simulink model "CAVE_MachE_speedTrack0202"  (R2019b)
settings: configuration reference "ConfigSetDesktopFixedStep" (kept outside this file)
PreLoadFcn:
  | VSS_BICYCLE=Simulink.Variant('Dual=0');
  | VSS_DUAL=Simulink.Variant('Dual=1');
  | Dual=1;
  | load('DriveCycle2.mat')
PostLoadFcn:
  | if any(exist('dsrtsu_mdlpostloadfcn', 'file') ~= 0), dsrtsu_mdlpostloadfcn('Execute', bdroot); end
InitFcn:
  | , if any(exist('dsmpb_private', 'file') ~= 0), dsmpb_private('dsmpb_mdlclblib', 'Init', bdroot); end,
  | load('DriveCycle2.mat')
model workspace (MAT data in the model file):
  Gas = 0.383333333333
values from neighbouring files (symbols this model uses):
  CoastDown =     [Run_Simulink.mat]
  limitedMCT =     [Run_Simulink.mat]
  MCT =     [Run_Simulink.mat]
  pMCT =     [Run_Simulink.mat]
  Ref_speed = [13 13.007895099 13.015778396 13.023649891 13.031509584 13.039357475 13.047193564 13.055017851 13.062830336 13.070631019 13.0784199 13.086196979 ... (2669 elements, 2669x1)]    [Ref_speed_and_time.mat]
  Ref_time = [0 0.01 0.02 0.03 0.04 0.05 0.06 0.07 0.08 0.09 0.1 0.11 ... (2669 elements, 2669x1)]    [Ref_speed_and_time.mat]
  US06 =     [Run_Simulink.mat]
undefined symbols (not defined in the file or in its folder): AccelCmd, ActTqLF_Nm_, ActTqLR_Nm_, ActTqRF_Nm_, ActTqRR_Nm_, BattChargeLimitMaxPwr, BattChargeLimitSocBpts, BattChargeLimitTbl, BattChrgCapcty, BattDischargeLimitSocBpts, BattDischargeLimitTbl, BattDischargeMaxPwr, BattNumCellsParallel, BattNumCellsSeries, BattOpenVoltCapBpts, BattOpenVoltTbl, BattResistSocBpts, BattResistTbl, BattResistTempBpts, BrakeMaxPrs, BrakeMaxTrq, ChassisDistCg2FrontAxle, ChassisDistCg2RearAxle, ChassisVehMass, CltchCmd, DecelCmd, DiffRatio, DiscIntNeverNeededParam, EnvGravCnst, EnvPrs, EnvTemp, FuelSpecificGrav, GearCmd, h, InitStates, lgSw, MtrEffSpdBpts, MtrEffTbl, MtrEffTrqBpts, MtrPwrMax, MtrTrqMax, Ref_Spd0229, Ref_Time0229, SteeringCmd, SupvsryCtrlRegenBrkCutOffTbl, SupvsryCtrlRegenSpdBpts, TestScnrioCycleNum, VEH
libraries: VSIGenLib x67, simulink x57, etargetslib x38, dsmpblib x28, vehdynlibtire x12, autolibshared x9, vehdynlibsuspension x7, vehdynlibtirecommon x7, autolibutils x5, CarMaker4SL x4, VsrLibWheel x4, autolibpowerinfoutils x3
(part 1 of 14)
PreSaveFcn:
  | , if any(exist('dsmpb_private', 'file') ~= 0), dsmpb_private('dsmpb_mdlclblib', 'PreSave', bdroot); end,
CloseFcn:
  | , if any(exist('dsmpb_private', 'file') ~= 0), dsmpb_private('dsmpb_mdlclblib', 'Close', bdroot); end,
settings Model: DataDictionary=DdPassengerEv.sldd  EnableAccessToBaseWorkspace=off  DSMPB_ID_DATA={'17923',struct('BlockId','31b0f37e-04c7-4ce1-8b16-8a1e9b5cfa15','SignalIds',{{'17c721c6-a3ae-4ad4-b238-642b1de755b7'}}),'17924',struct('BlockId','bcfd9437-88e4-4cd6-b7b0-947b12d9129e','SignalIds',{{'e279c9ec-6196-4878-b889-71a854f53d02'}}),'17925',struct('BlockId','c62c3796-2ab1-49a7-b1e5-4d980e0bcb0b','SignalIds',{{'f66872c7-5266-4e77-ba9d-87065806d94f'}}),'17926',struct('BlockId','40b2dd3c-dc50-4d54-adc2-8ba9b18f36d5','SignalIds',{{'523e7fc5-5d31-4807-939d-dbbffd70444f'}}),'17927',struct('BlockId','e8d674f4-c081-4c3a-b2b1-2d0ab8133194','SignalIds',{{'0eda9826-4c02-4cc0-9f18-cf69c46de25a','ab39894a-9bf0-4e2b-9c49-db18f6b4bbcb','ed4e635a-610c-4130-b876-996df8d6f23e','d7b08fa0-5164-4c6c-899c-f7c626698d6c','66095545-3d28-434a-a0e8-d46feba78e3b'}}),'17928',struct('BlockId','74aeb7d1-659c-488e-9138-a7590a989d80','SignalIds',{{'26f36065-db9f-4eb5-8bd7-2ab8ed1530af','9b8b33d1-0c3b-4425-9130-99ff6edfa98a'}}),'17929',struct('BlockId','1e8a7d48-41ff-4223-b4b4-ccd9c4207a27','SignalIds',{{'1b0cf8dd-8605-4169-a6de-39231325f0e5'}}),'17935',struct('BlockId','a5f9a6b1-85ee-410c-8934-50052dbd8ca7','SignalIds',{{'ba3b2526-034b-43f6-a555-dff2bea2cc85'}}),'17936',struct('BlockId','1e1892f8-2999-45dd-a8da-0e8121fc388b','SignalIds',{{'4c47874d-0703-4ff1-9abe-c2ce178ef0a7'}}),'17937',struct('BlockId','e85c17ff-dd30-482c-995d-c0a74f106bb8','SignalIds',{{'8160658a-6bed-4f87-b995-d0b653e3718e'}}),'17938',struct('BlockId','e3071f67-61ca-4ccc-876b-23b50e94809a','SignalIds',{{'03fc8176-d730-4c60-914d-7ce6c370162b'}}),'17939',struct('BlockId','6cc6af10-99b5-45df-ab2c-9d119c31698c','SignalIds',{{'65b90dff-5318-4540-88c9-38859f061b45'}}),'17940',struct('BlockId','0db74d10-8518-4861-b223-fb8645ae7c50','SignalIds',{{'f8b55a51-0374-486e-9c03-7d81119e1378'}}),'17941',struct('BlockId','43054e70-1d94-41e4-ae6d-92ba2dcfefa2','SignalIds',{{'310153da-09e7-4a32-aa01-e5bac30a61fd'}}),'17942',struct('BlockId','d4d6f3b7-e9bb-4bfb-ad6d-7b0539ed1dac','SignalIds',{{'32f338f5-3495-4abe-a586-ce83ab37ca6d'}}),'18088',struct('BlockId','f88c42c2-e70e-4436-bd85-ff34452e836e','SignalIds',{{'1df572a0-f117-4729-9091-2c1a0a26ec90','0824b86c-995c-4624-95de-4f5a118cf0f7','1af539eb-325a-4e38-9107-84d6b0267392','ebb0fa34-559f-4fe0-b409-8a817ae8753c','d7145080-d35d-4c02-8c9e-cf76ffb14dc2','5075bfde-4142-4aeb-b309-025b37120541','abbab0bd-1456-4252-a37b-ee5f55ea0579','b5d617b8-bb24-4539-9145-e591a0a295f8','7df03788-1936-4801-98c0-dd7f6dfcacba','19949bfb-f246-4995-90e8-29a3751a0fa7','9454b59a-aedd-4270-89a6-1cca43305823','37cf720c-23c2-4b6d-8589-7b035c806643','98db9f76-eafd-4d54-90d2-d997d73b87d4','ff589fc8-5b21-4798-a75e-d26fc35c1fa1','e61b2882-e27e-4f06-b730-5e5281621b34','6605e0e6-8bf3-4a45-a0b0-4b9c1cf463f3','0d0f5161-daad-47a1-bb1d-ec2adbc183ca','48ba6675-0966-4a1c-b127-4f76dca3de94','3c897f11-b2eb-4eb8-b88f-7b7e913c6e41','378f468e-364f-43c5-91f9-fc8ddef6aca6','9c7f20ac-956d-4c19-bdea-31a2a3930ea2','bc252920-9c7c-4b91-a017-ee1d69e3f03c','a5e7a104-8664-4690-a58a-7cbf05737866','fe1cfa34-9b23-4225-85e3-0403f07d36e7','ab40d80a-815e-4994-aacd-e42d283f5b3a','2a4143b2-c438-4d42-997d-0587141eb8f0','2686c37a-8724-40b3-99fb-f8873ba286b8','3707aa1b-88c1-4f14-8f25-f346aa75c252','7413af4b-f834-4020-ad34-3dd98c546e0c','3445835b-9a90-4408-a32d-d76b66b0385b','23c9a144-1259-4fa3-9a16-4a32a7eadff9','5b4206b0-ea89-4111-86f7-7a4fd8c76b72','85c84ea6-72b6-4ccb-9199-727b305580c3','97bb0073-9d03-44a9-972d-49a0eb465678','8c3f0698-b0b6-4624-aa00-3a3096f7cc2f','c968922f-253e-433f-ad46-daf21e902962','21ad150a-19dc-415b-bc1b-b39528ec9221','a3572415-9467-4ff8-a492-c6c1b3cb1b64','700ac678-fb53-40b6-8e97-9eeffe7a1ca8','14ed5f8b-aa1d-402b-b493-5622a729893d','bdbcc0b3-c6a4-485e-8fbf-8c12a8df89e7','7a19cc2b-f06b-466f-ae52-fb8ac6fb0258','87deda6a-2251-4462-8ae0-a20845c776d4','41874d9b-304a-4265-a3a1-69d5c58383ea'}}),'18175',struct('BlockId','8445dc7e-f46b-4bf1-918c-6ff4bf4b4269','SignalIds',{{'24a6103b-da21-4c61-bcdd-b18edd3e31e0'}}),'18251',struct('BlockId','87dadb4f-598f-4630-a764-aa9dbd54dbe2','SignalIds',{{'83e82515-562b-4cea-9022-e0067df93a7f','d6888abe-93df-4986-aa37-664290aa1833','c6c9ff24-fc0f-4a39-be02-e6acd6045705','d4d14bee-f141-4067-bca8-9bf015562c80','1613add9-a5cb-4969-b219-0bfd270ce741'}}),'18719',struct('BlockId','79daabbd-4df4-4017-ba65-d977f7e6cd2f','SignalIds',{{'63c99320-3a8a-469e-8a50-5c577229603f'}}),'18720',struct('BlockId','9f21d727-31d5-41b9-aed1-27a40d8edf8b','SignalIds',{{'abab19c9-0d91-46eb-acba-2a4710e305d8'}}),'18721',struct('BlockId','5513e588-accc-447f-8233-209349c29c53','SignalIds',{{'cf7c35a9-6bda-4f5f-bfb5-f51ad44c376b'}}),'18722',struct('BlockId','a427ee23-ff95-4a9c-807f-ad2b61c33ee4','SignalIds',{{'b3e368f1-9670-4dd7-aa42-1fcccca64ddf'}}),'18723',struct('BlockId','53805a71-03ad-4b45-a2ab-66e4ec3700d0','SignalIds',{{'0801da20-d997-46db-8512-e37e1180e77c','d193450d-1a5a-4c8d-a2ac-d5fd306fefe3'}}),'18724',struct('BlockId','4d4909f9-4869-4ae2-8541-060fc5e29366','SignalIds',{{'0588d1ac-5d02-4ce0-9f56-5f4e572c1088','c0609b3e-104e-46bb-beb6-dc1d54d218ce','a0011887-c3f0-4769-95be-c916ccb77447','feb7a80d-e7d1-407d-8b44-49f086fb9d8a'}}),'19413',struct('BlockId','0cb03894-8e97-4ee1-8e6b-a64372051d89','SignalIds',{{'fb9cdb0d-760c-44d1-8213-f9fd5c714171'}}),'19414',struct('BlockId','a8b270f5-6693-4c61-9523-aedd8553eba8','SignalIds',{{'ee97cdc8-c0b4-47f5-b123-39b38da02150','8741976f-1948-4d6a-bb05-1c8ff31e49c6','e35d9971-1b34-4271-b70b-fcd309649aaa','85271c6c-839f-44b8-900d-ba9a8fe0ef7f','0bee37df-31a4-417c-8557-0974603250da'}}),'19415',struct('BlockId','d1b05c0a-1ae7-443d-b188-dcb43e72f6c3','SignalIds',{{'5e73da08-5070-4b81-9c98-37bbd0e992f4','72282e92-6e64-45e0-b1f8-4355a24ba605'}}),'19416',struct('BlockId','eeda17f4-d85b-4dfd-9f8d-73f45548cecc','SignalIds',{{'2351cc6d-fd94-414e-86e0-ed4604027b49'}})}  RTICANMMDATA=struct('GeneralSetupData',struct('modelroot','C:\GitDev\Anye\cave_carla_dev\Vehicles\VehicleProjects\Bolt_EV\System','generalsettings',struct('filesettings',struct('destfolder',struct('Name','RTICANMM_FILES','Check',1),'buildfolder',struct('Name','.','Check',1),'AbsDestfolder',struct('Name','C:\GitDev\Anye\cave_carla_dev\Vehicles\VehicleProjects\Bolt_EV\System\RTICANMM_FILES'),'AbsBuildfolder',struct('Name','C:\GitDev\Anye\cave_carla_dev\Vehicles\VehicleProjects\Bolt_EV\System'))),'options',struct('addpaths',1,'rmpaths',1,'addtrcexclusion',true,'cannavigator',struct('checkmonitoring',0),'show_usrtrc',0,'use_usrtrc',0),'advanced',struct('options',ones(1,100)),'MPSetup',{{}},'RTI',struct('Type','DSRT','Ver','4.2p1','Date','11-Feb-2020'),'modelname','CAVE_MachE_speedTrack0202','block','CAVE_MachE_speedTrack0202'))  DSRTSU_INTERNAL_RTIFPGA=150  PauseTimes=45  EnablePacing=on  OrderedModelArguments=off  Creator=9bt  LastModifiedBy=RVDP
settings ConfigSetRef: SourceName=ConfigSetDesktopFixedStep

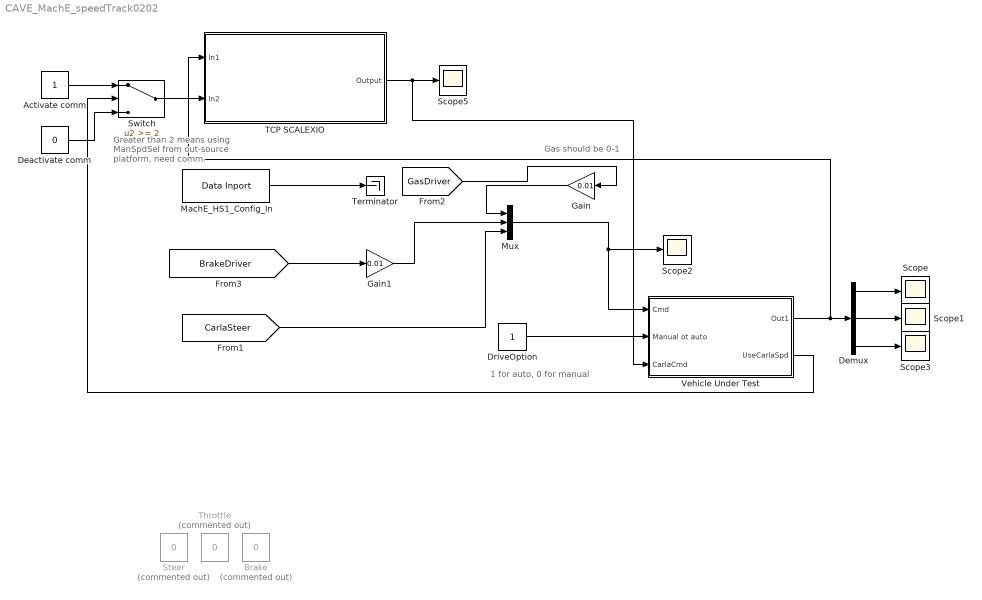
== system CAVE_MachE_speedTrack0202 ==
  note: Greater than 2 means using ManSpdSel from out-source platform, need comm.
  note: 1 for auto, 0 for manual
  note: Gas should be 0-1
  Activate comm : Constant
  Brake : Constant  Commented=on  Value=0
  Deactivate comm : Constant  Value=0
  Demux : Demux  Outputs=5
  DriveOption : Constant
  Gain : Gain  Gain=0.01
  Gain1 : Gain  Gain=0.01
  MachE_HS1_Config_In : dsmpblib/Data Inport  Priority=10000
      settings: SourceProductName=dSPACE Model Interface Blockset
  Mux : Mux  Inputs=3
  Scope{,1..3,5} (5 alike) : Scope
  Steer : Constant  Commented=on  Value=0
  Switch : Switch  Threshold=2
  TCP SCALEXIO : Subsystem
  Terminator : Terminator
  Throttle : Constant  Commented=on  Value=0
  Vehicle Under Test : Subsystem
  wires:
  Demux/1 -> Scope/1
  Mux/1 -> Vehicle Under Test/1(Cmd), Scope2/1
  Demux/3 -> Scope1/1
  DriveOption/1 -> Vehicle Under Test/2(Manual ot auto)
  [GasDriver] -> Gain/1
  [BrakeDriver] -> Gain1/1
  MachE_HS1_Config_In/1 -> Terminator/1
  Gain/1 -> Mux/1
  Gain1/1 -> Mux/2
  Vehicle Under Test/1(Out1) -> TCP SCALEXIO/1(In1), Demux/1
  Switch/1 -> TCP SCALEXIO/2(In2)
  TCP SCALEXIO/1(Output) -> Vehicle Under Test/3(CarlaCmd), Scope5/1
  Demux/5 -> Scope3/1
  Deactivate comm/1 -> Switch/3
  Activate comm/1 -> Switch/1
  Vehicle Under Test/2(UseCarlaSpd) -> Switch/2
  [CarlaSteer] -> Mux/3

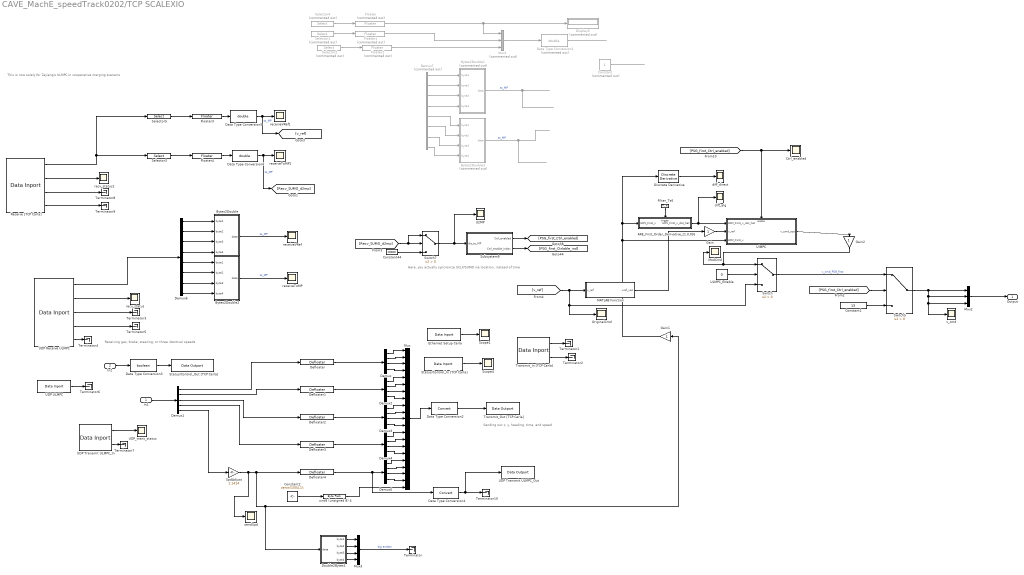
== system CAVE_MachE_speedTrack0202/TCP SCALEXIO ==
  note: This is now solely for Zejiang's ULMPC in cooperative merging scenario
  note: Receiving gas, brake, steering; or three identical speeds
  note: Sending out x, y, heading, time, and speed
  note: Here, you actually syncronize SCLX/SUMO via location, instead of time
  In1 : Inport
  In2 : Inport  Port=2
  ARE_First_Order_Derivative_[1,0,0]6 : Subsystem  TreatAsAtomicUnit=on
  Bytes2Double : Subsystem
  Bytes2Double1 : Subsystem  Commented=on
  Bytes2Double2 : Subsystem
  Bytes2Double3 : Subsystem  Commented=on
  Constant : Constant  Commented=on  OutDataTypeStr=boolean
  Constant1 : Constant  Value=13
  Constant2 : Constant  Value=zeros(1004,1);  OutDataTypeStr=uint8
  Constant44 : Constant  Value=10000
  Ctrl_enabled : Scope
  Data Type Conversion1 : DataTypeConversion  Commented=on  OutDataTypeStr=double
  Data Type Conversion2 : DataTypeConversion
  Data Type Conversion3 : DataTypeConversion  OutDataTypeStr=boolean
  Data Type Conversion4 : DataTypeConversion
  Data Type Conversion5 : DataTypeConversion  OutDataTypeStr=double
  Data Type Conversion6 : DataTypeConversion  OutDataTypeStr=double
  Defloater{,1..4} (5 alike) : VSIGenLib/Defloater  SystemSampleTime=-1  Latency=0  AutoFrameSizeCalculation=off
  Demux{,2..5} (5 alike) : Demux
  Demux1 : Demux  Outputs=5
  Demux6 : Demux  Outputs=8
  Demux7 : Demux  Commented=on  Outputs=8
  Discrete Derivative : simulink/Discrete/Discrete Derivative  gainval=1.0  ICPrevScaledInput=0.0  OutMin=[]  OutMax=[]  OutDataType=fixdt(1, 16)  OutScaling=2^-10  DoSatur=off
  Display3 : Display  Commented=on
  Double2Bytes1 : Subsystem
  Ethernet Setup Carla : dsmpblib/Data Inport  Priority=10000
      settings: SourceProductName=dSPACE Model Interface Blockset
  Filter_Ts6 : DiscretePulseGenerator  PulseType=Time based  Period=0.01*2  PulseWidth=50
  Floater : VSIGenLib/Floater  Commented=on  SystemSampleTime=-1  Latency=0  AutoFrameSizeCalculation=off
  Floater1 : VSIGenLib/Floater  Commented=on  SystemSampleTime=-1  Latency=0  AutoFrameSizeCalculation=off
  Floater2 : VSIGenLib/Floater  Commented=on  SystemSampleTime=-1  Latency=0  AutoFrameSizeCalculation=off
  Floater3 : VSIGenLib/Floater  SystemSampleTime=-1  Latency=0  AutoFrameSizeCalculation=off
  Floater4 : VSIGenLib/Floater  SystemSampleTime=-1  Latency=0  AutoFrameSizeCalculation=off
  Gain : Gain
  Gain1 : Gain
  Gain2 : Gain
  MATLAB Function : MATLAB Function  TreatAsAtomicUnit=on
  ModCmd : Scope
  Mux : Mux  Inputs=21
  Mux1 : Mux  Commented=on  Inputs=3
  Mux2 : Mux  Inputs=3
  Mux3 : Mux
  OriginalCmd : Scope
  Receive [TCP Carla] : dsmpblib/Data Inport  Priority=10000
      settings: SourceProductName=dSPACE Model Interface Blockset
  Scope1 : Scope
  Scope4 : Scope
  Selector1 : Selector  Commented=on  InputPortWidth=1024  IndexOptions=Index vector (dialog)  Indices=[8 7 6 5]  OutputSizes=1
  Selector2 : Selector  Commented=on  InputPortWidth=1024  IndexOptions=Index vector (dialog)  Indices=[12 11 10 9]  OutputSizes=1
  Selector3 : Selector  InputPortWidth=8  IndexOptions=Index vector (dialog)  Indices=[8 7 6 5]  OutputSizes=1
  Selector4 : Selector  Commented=on  InputPortWidth=1024  IndexOptions=Index vector (dialog)  Indices=[4 3 2 1]  OutputSizes=1
  Selector5 : Selector  InputPortWidth=8  IndexOptions=Index vector (dialog)  Indices=[4 3 2 1]  OutputSizes=1
  SpdAdjust : Gain  Gain=1.1414
  Status/Control_In [TCP Carla] : dsmpblib/Data Inport  Priority=10000
      settings: SourceProductName=dSPACE Model Interface Blockset
  Status/Control_Out [TCP Carla] : dsmpblib/Data Outport  Priority=-10000
      settings: SourceProductName=dSPACE Model Interface Blockset
  Subsystem9 : Subsystem
  Switch : Switch  Criteria=u2 > Threshold
  Switch5 : Switch  Criteria=u2 > Threshold
  Switch7 : Switch  Criteria=u2 > Threshold
  Terminator{,1..10} (11 alike) : Terminator
  Transmit_In [TCP Carla] : dsmpblib/Data Inport  Priority=10000
      settings: SourceProductName=dSPACE Model Interface Blockset
  Transmit_Out [TCP Carla] : dsmpblib/Data Outport  Priority=-10000
      settings: SourceProductName=dSPACE Model Interface Blockset
  UDP Receive ULMPC : dsmpblib/Data Inport  Priority=10000
      settings: SourceProductName=dSPACE Model Interface Blockset
  UDP Transmit ULMPC_In : dsmpblib/Data Inport  Priority=10000
      settings: SourceProductName=dSPACE Model Interface Blockset
  UDP Transmit ULMPC_Out : dsmpblib/Data Outport  Priority=-10000
      settings: SourceProductName=dSPACE Model Interface Blockset
  UDP ULMPC : dsmpblib/Data Inport  Priority=10000
      settings: SourceProductName=dSPACE Model Interface Blockset
  UDP_trans_status : Scope
  ULMPC_ENable : Constant  Value=0  OutDataTypeStr=Inherit: Inherit via back propagation
  UlMPC : Subsystem
  d2MP : Scope
  diff_alg : Scope
  diff_direct : Scope
  receiveToMP : Scope
  receiveToMP1 : Scope
  receiveVRef : Scope
  receiveVRef1 : Scope
  recv_status : Scope
  recv_status1 : Scope
  sendSpd : Scope
  uint8 (unsigned 8) 4 : etargetslib/Byte Pack  datatypes={'uint8'}  byteAlign=1
      settings: SourceProductName=MATLAB Coder
  v_cmd : Scope
  Output : Outport
  wires:
  Demux4/4 -> Mux/16
  Demux3/4 -> Mux/12
  Defloater1/1 -> Demux2/1
  Mux/1 -> Data Type Conversion2/1
  Demux4/2 -> Mux/14
  Demux3/1 -> Mux/9
  Demux/4 -> Mux/4
  Demux/1 -> Mux/1
  Demux2/4 -> Mux/8
  Demux1/3 -> Defloater2/1
  Defloater/1 -> Demux/1
  Defloater3/1 -> Demux4/1
  Demux3/3 -> Mux/11
  Demux1/2 -> Defloater1/1
  Demux2/2 -> Mux/6
  Constant2/1 -> uint8 (unsigned 8) 4/1
  Demux1/1 -> Defloater/1
  Defloater2/1 -> Demux3/1
  Demux1/4 -> Defloater3/1
  Demux3/2 -> Mux/10
  Demux/3 -> Mux/3
  Demux/2 -> Mux/2
  In1/1 -> Demux1/1
  Demux2/1 -> Mux/5
  Demux4/1 -> Mux/13
  Demux2/3 -> Mux/7
  Demux4/3 -> Mux/15
  Transmit_In [TCP Carla]/2 -> Terminator2/1
  Transmit_In [TCP Carla]/1 -> Terminator1/1
  UDP Receive ULMPC/2 -> recv_status/1
  Data Type Conversion3/1 -> Status/Control_Out [TCP Carla]/1
  In2/1 -> Data Type Conversion3/1
  UDP Receive ULMPC/4 -> Terminator5/1
  UDP Receive ULMPC/3 -> Terminator3/1
  Status/Control_In [TCP Carla]/1 -> Scope4/1
  Ethernet Setup Carla/1 -> Scope1/1
  Demux1/5 -> SpdAdjust/1
  Demux5/2 -> Mux/18
  Demux5/3 -> Mux/19
  Demux5/4 -> Mux/20
  uint8 (unsigned 8) 4/1 -> Mux/21
  Demux5/1 -> Mux/17
  Defloater4/1 -> Data Type Conversion4/1, Demux5/1
  Data Type Conversion2/1 -> Transmit_Out [TCP Carla]/1
  Discrete Derivative/1 -> diff_direct/1
  Gain2/1 -> ModCmd/1, Switch/1
  Gain/1 -> UlMPC/2(v_ref)
  UlMPC/1(v_cmd_opt) -> Gain2/1
  ULMPC_ENable/1 -> Switch/2
  Gain1/1 -> Discrete Derivative/1, ARE_First_Order_Derivative_[1,0,0]6/1(HDV_First_v), UlMPC/3(HDV_First_v)
  ARE_First_Order_Derivative_[1,0,0]6/1(HDV_First_v_dot_hat) -> diff_alg/1, UlMPC/1(HDV_First_v_dot_hat)
  Filter_Ts6/1 -> ARE_First_Order_Derivative_[1,0,0]6/Trigger
  Constant44/1 -> Switch7/3
  Switch7/1 -> d2MP/1, Subsystem9/1(dis_to_MP)
  Subsystem9/2(Ctrl_enable_Index) -> [PSG_first_Ctrlable_ind]
  [Recv_SUMO_d2mp] -> Switch7/1, Switch7/2
  [v_ref] -> Switch/3, OriginalCmd/1, MATLAB Function/1(v_ref)
  MATLAB Function/1(vref_vec) -> Gain/1
  [PSG_first_Ctrl_enabled] -> Ctrl_enabled/1, UlMPC/Enable
  [PSG_first_Ctrl_enabled] -> Switch5/2
  Constant1/1 -> Switch5/3
  Switch/1 -> Switch5/1  "v_cmd_PSG_first"
  Selector1/1 -> Floater1/1
  Selector4/1 -> Floater/1
  ? -> Selector4/1, Selector2/1, Selector1/1
  Floater/1 -> Display3/1, Mux1/1
  Floater2/1 -> Mux1/3
  Mux1/1 -> Data Type Conversion1/1
  Data Type Conversion1/1 -> ?
  Selector2/1 -> Floater2/1
  Floater1/1 -> Mux1/2
  Switch5/1 -> Mux2/1, Mux2/2, Mux2/3, v_cmd/1
  Mux2/1 -> Output/1
  Demux6/1 -> Bytes2Double/1(byte1)
  Demux6/3 -> Bytes2Double/3(byte3)
  Demux6/5 -> Bytes2Double2/1(byte1)
  Demux6/6 -> Bytes2Double2/2(byte2)
  Demux6/8 -> Bytes2Double2/4(byte4)
  Demux6/7 -> Bytes2Double2/3(byte3)
  Demux6/4 -> Bytes2Double/4(byte4)
  Demux6/2 -> Bytes2Double/2(byte2)
  UDP Receive ULMPC/5 -> Terminator4/1
  UDP ULMPC/1 -> Terminator6/1
  UDP Transmit ULMPC_In/1 -> UDP_trans_status/1
  UDP Transmit ULMPC_In/2 -> Terminator7/1
  UDP Receive ULMPC/1 -> Demux6/1
  Receive [TCP Carla]/4 -> Terminator9/1
  Receive [TCP Carla]/3 -> Terminator8/1
  Receive [TCP Carla]/2 -> recv_status1/1
  SpdAdjust/1 -> sendSpd/1, Defloater4/1, Double2Bytes1/1(data), Gain1/1
  Double2Bytes1/3(byte3) -> Mux3/3
  Double2Bytes1/2(byte2) -> Mux3/2
  Double2Bytes1/1(byte1) -> Mux3/1
  Double2Bytes1/4(byte4) -> Mux3/4
  Data Type Conversion4/1 -> Terminator10/1, UDP Transmit ULMPC_Out/1
  Mux3/1 -> Terminator/1  "big endian"
  Constant/1 -> ?
  Floater3/1 -> Data Type Conversion5/1
  Selector5/1 -> Floater3/1
  Floater4/1 -> Data Type Conversion6/1
  Selector3/1 -> Floater4/1
  Bytes2Double2/1(data) -> receiveToMP/1  "to_MP"
  Bytes2Double/1(data) -> receiveVRef/1  "to_MP"
  Demux7/6 -> Bytes2Double3/2(byte2)
  Bytes2Double3/1(data) -> ?  "to_MP"
  Demux7/1 -> Bytes2Double1/1(byte1)
  Demux7/5 -> Bytes2Double3/1(byte1)
  Bytes2Double1/1(data) -> ?  "to_MP"
  Demux7/3 -> Bytes2Double1/3(byte3)
  Demux7/2 -> Bytes2Double1/2(byte2)
  Demux7/4 -> Bytes2Double1/4(byte4)
  Demux7/7 -> Bytes2Double3/3(byte3)
  Demux7/8 -> Bytes2Double3/4(byte4)
  ? -> Demux7/1
  Receive [TCP Carla]/1 -> Selector3/1, Selector5/1
  Data Type Conversion5/1 -> [v_ref], receiveVRef1/1  "to_MP"
  Data Type Conversion6/1 -> [Recv_SUMO_d2mp], receiveToMP1/1  "to_MP"
  Subsystem9/1(Ctrl_enabled) -> [PSG_first_Ctrl_enabled]

== system CAVE_MachE_speedTrack0202/Vehicle Under Test ==
  Cmd : Inport
  Manual ot auto : Inport  Port=2
  CarlaCmd : Inport  Port=3
  AccelCmdOutput_Anye : Terminator
  Ackerman steer : Lookup_n-D  NumberOfTableDimensions=1  BreakpointsForDimension1="[-0.446316297916244\t-0.442150786830951\t-0.437977161945005\t-0.433795286969319\t-0.429605025209166\t-0.425406239561593\t-0.421198792513030\t-0.416982546137136\t-0.412757362092861\t-0.408523101622746\t-0.404279625551461\t-0.400026794284603\t-0.395764467807732\t-0.391492505685692\t-0.387210767062193\t-0.382919110659678\t-0.378617394779480\t-0.374305477302279\t-0.369983215688866\t-0.365650466981227\t-0.361307087803951\t-0.356952934365975\t-0.352587862462675\t-0.348211727478321\t-0.343824384388886\t-0.339425687765245\t-0.335015491776758\t-0.330593650195247\t-0.326160016399396\t-0.321714443379563\t-0.317256783743034\t-0.312786889719717\t-0.308304613168298\t-0.303809805582871\t-0.299302318100048\t-0.294782001506567\t-0.290248706247410\t-0.285702282434450\t-0.281142579855627\t-0.276569447984685\t-0.271982735991464\t-0.267382292752788\t-0.262767966863931\t-0.258139606650706\t-0.253497060182174\t-0.248840175283994\t-0.244168799552432\t-0.239482780369037\t-0.234781964916014\t-0.230066200192295\t-0.225335333030331\t-0.220589210113630\t-0.215827677995039\t-0.211050583115807\t-0.206257771825433\t-0.201449090402323\t-0.196624385075265\t-0.191783502045761\t-0.186926287511198\t-0.182052587688919\t-0.177162248841170\t-0.172255117300976\t-0.167331039498945\t-0.162389861991014\t-0.157431431487183\t-0.152455594881217\t-0.147462199281363\t-0.142451092042095\t-0.137422120796894\t-0.132375133492088\t-0.127309978421782\t-0.122226504263869\t-0.117124560117169\t-0.112003995539695\t-0.106864660588066\t-0.101706405858090\t-0.0965290825265349\t-0.0913325423940914\t-0.0861166379295599\t-0.0808812223152671\t-0.0756261494937309\t-0.0703512742155897\t-0.0650564520888085\t-0.0597415396291770\t-0.0544063943121130\t-0.0490508746257825\t-0.0436748401255510\t-0.0382781514897739\t-0.0328606705769398\t-0.0274222604841732\t-0.0219627856071077\t-0.0164821117011354\t-0.0109801059440403\t-0.00545663700002112\t0\t0.00547767577609933\t0.0110656090794470\t0.0166755107772618\t0.0223075038233658\t0.0279617092740365\t0.0336382462142580\t0.0393372316825870\t0.0450587805946413\t0.0508030056652199\t0.0565700173290652\t0.0623599236602815\t0.0681728302904245\t0.0740088403252790\t0.0798680542603446\t0.0857505698950509\t0.0916564822457268\t0.0975858834573503\t0.103538862714108\t0.109515506148794\t0.115515896751090\t0.121540114274751\t0.127588235143750\t0.133660332357415\t0.139756475394610\t0.145876730117007\t0.152021158671496\t0.158189819391799\t0.164382766699339\t0.170600051003425\t0.176841718600822\t0.183107811574771\t0.189398367693541\t0.195713420308563\t0.202052998252265\t0.208417125735647\t0.214805822245717\t0.221219102442855\t0.227656976058216\t0.234119447791246\t0.240606517207442\t0.247118178636427\t0.253654421070478\t0.260215228063589\t0.266800577631217\t0.273410442150791\t0.280044788263140\t0.286703576774936\t0.293386762562311\t0.300094294475738\t0.306826115246357\t0.313582161393837\t0.320362363135953\t0.327166644299990\t0.333994922236136\t0.340847107733006\t0.347723104935443\t0.354622811264752\t0.361546117341510\t0.368492906911125\t0.375463056772267\t0.382456436708368\t0.389472909422305\t0.396512330474460\t0.403574548224288\t0.410659403775562\t0.417766730925451\t0.424896356117582\t0.432048098399246\t0.439221769382891\t0.446417173212069\t0.453634106531970\t0.460872358464695\t0.468131710589418\t0.475411936927561\t0.482712803933137\t0.490034070488372\t0.497375487904758\t0.504736799929627\t0.512117742758400\t0.519518045052588\t0.526937427963674\t0.534375605162959\t0.541832282877473\t0.549307159932028\t0.556799927797496\t0.564310270645373\t0.571837865408689\t0.579382381849329\t0.586943482631776\t0.594520823403350\t0.602114052880920\t0.609722812944144\t0.617346738735206\t0.624985458765058]"  Table="[-9.40000000000000\t-9.30000000000000\t-9.20000000000000\t-9.10000000000000\t-9\t-8.90000000000000\t-8.80000000000000\t-8.70000000000000\t-8.60000000000000\t-8.50000000000000\t-8.40000000000000\t-8.30000000000000\t-8.20000000000000\t-8.10000000000000\t-8\t-7.90000000000000\t-7.80000000000000\t-7.70000000000000\t-7.60000000000000\t-7.50000000000000\t-7.40000000000000\t-7.30000000000000\t-7.20000000000000\t-7.10000000000000\t-7\t-6.90000000000000\t-6.80000000000000\t-6.70000000000000\t-6.60000000000000\t-6.50000000000000\t-6.40000000000000\t-6.30000000000000\t-6.20000000000000\t-6.10000000000000\t-6\t-5.90000000000000\t-5.80000000000000\t-5.70000000000000\t-5.60000000000000\t-5.50000000000000\t-5.40000000000000\t-5.30000000000000\t-5.20000000000000\t-5.10000000000000\t-5\t-4.90000000000000\t-4.80000000000000\t-4.70000000000000\t-4.60000000000000\t-4.50000000000000\t-4.40000000000000\t-4.30000000000000\t-4.20000000000000\t-4.10000000000000\t-4\t-3.90000000000000\t-3.80000000000000\t-3.70000000000000\t-3.60000000000000\t-3.50000000000000\t-3.40000000000000\t-3.30000000000000\t-3.20000000000000\t-3.10000000000000\t-3\t-2.90000000000000\t-2.80000000000000\t-2.70000000000000\t-2.60000000000000\t-2.50000000000000\t-2.40000000000000\t-2.30000000000000\t-2.20000000000000\t-2.10000000000000\t-2\t-1.90000000000000\t-1.80000000000000\t-1.70000000000000\t-1.60000000000000\t-1.50000000000000\t-1.40000000000000\t-1.30000000000000\t-1.20000000000000\t-1.10000000000000\t-1\t-0.900000000000000\t-0.800000000000000\t-0.700000000000000\t-0.600000000000000\t-0.500000000000000\t-0.400000000000000\t-0.300000000000000\t-0.200000000000000\t-0.100000000000000\t0\t0.100000000000000\t0.200000000000000\t0.300000000000000\t0.400000000000000\t0.500000000000000\t0.600000000000000\t0.700000000000000\t0.800000000000000\t0.900000000000000\t1\t1.10000000000000\t1.20000000000000\t1.30000000000000\t1.40000000000000\t1.50000000000000\t1.60000000000000\t1.70000000000000\t1.80000000000000\t1.90000000000000\t2\t2.10000000000000\t2.20000000000000\t2.30000000000000\t2.40000000000000\t2.50000000000000\t2.60000000000000\t2.70000000000000\t2.80000000000000\t2.90000000000000\t3\t3.10000000000000\t3.20000000000000\t3.30000000000000\t3.40000000000000\t3.50000000000000\t3.60000000000000\t3.70000000000000\t3.80000000000000\t3.90000000000000\t4\t4.10000000000000\t4.20000000000000\t4.30000000000000\t4.40000000000000\t4.50000000000000\t4.60000000000000\t4.70000000000000\t4.80000000000000\t4.90000000000000\t5\t5.10000000000000\t5.20000000000000\t5.30000000000000\t5.40000000000000\t5.50000000000000\t5.60000000000000\t5.70000000000000\t5.80000000000000\t5.90000000000000\t6\t6.10000000000000\t6.20000000000000\t6.30000000000000\t6.40000000000000\t6.50000000000000\t6.60000000000000\t6.70000000000000\t6.80000000000000\t6.90000000000000\t7\t7.10000000000000\t7.20000000000000\t7.30000000000000\t7.40000000000000\t7.50000000000000\t7.60000000000000\t7.70000000000000\t7.80000000000000\t7.90000000000000\t8\t8.10000000000000\t8.20000000000000\t8.30000000000000\t8.40000000000000\t8.50000000000000\t8.60000000000000\t8.70000000000000\t8.80000000000000\t8.90000000000000\t9\t9.10000000000000\t9.20000000000000\t9.30000000000000\t9.40000000000000]"  InternalRulePriority=Speed  RndMeth=Simplest  InputSameDT=on
  Bus Creator : BusCreator  Inputs=AccelCmd,DecelCmd,GearCmd,CltchCmd,lgSw,SteeringCmd
  Bus Creator1 : BusCreator  Inputs=8
  Bus Creator2 : BusCreator  Inputs=2
  Bus Selector : BusSelector  OutputSignals=Veh.Chassis.X,Veh.Chassis.Y,Veh.Chassis.psi,Veh.Batt.BattSoc,Veh.Batt.BattCurr,Veh.Batt.BattVolt,Veh.Diff.Axl1.Axl1Trq,Veh.Chassis.VehSpd
  Clock : Clock
  Constant : Constant  Value=0
  Constant2 : Constant
  Constant3 : Constant  Value=0
  Constant4 : Constant
  Constant6 : Constant  Value=0.5  SampleTime=-1
  Demux : Demux  Outputs=3
  EV Bolt Steer : Lookup_n-D  NumberOfTableDimensions=1  BreakpointsForDimension1="[-0.541571931581492\t-0.535619550629112\t-0.529667169676731\t-0.523714788724350\t-0.517762407771969\t-0.511810026819588\t-0.505857645867207\t-0.499905264914826\t-0.493952883962445\t-0.488000503010064\t-0.482048122057683\t-0.476095741105302\t-0.470143360152921\t-0.464190979200541\t-0.458238598248160\t-0.452286217295779\t-0.446333836343398\t-0.440381455391017\t-0.434429074438636\t-0.428476693486255\t-0.422524312533874\t-0.416571931581493\t-0.410619550629112\t-0.404667169676731\t-0.398714788724350\t-0.392762407771969\t-0.386810026819588\t-0.380857645867207\t-0.374905264914826\t-0.368952883962445\t-0.363000503010064\t-0.357048122057683\t-0.351095741105302\t-0.345143360152921\t-0.339190979200541\t-0.333238598248160\t-0.327286217295779\t-0.321333836343398\t-0.315381455391017\t-0.309429074438636\t-0.303476693486255\t-0.297524312533874\t-0.291571931581493\t-0.285619550629112\t-0.279667169676731\t-0.273714788724350\t-0.267762407771969\t-0.261810026819588\t-0.255857645867207\t-0.249905264914826\t-0.243952883962445\t-0.238000503010065\t-0.232048122057684\t-0.226095741105303\t-0.220143360152922\t-0.214190979200541\t-0.208238598248160\t-0.202286217295779\t-0.196333836343398\t-0.190381455391017\t-0.184429074438636\t-0.178476693486255\t-0.172524312533874\t-0.166571931581493\t-0.160619550629112\t-0.154667169676731\t-0.148714788724350\t-0.142762407771969\t-0.136810026819588\t-0.130857645867207\t-0.124905264914826\t-0.118952883962445\t-0.113000503010064\t-0.107048122057683\t-0.101095741105303\t-0.0951433601529216\t-0.0891909792005406\t-0.0832385982481596\t-0.0772862172957787\t-0.0713338363433977\t-0.0653814553910168\t-0.0594290744386358\t-0.0534766934862548\t-0.0475243125338739\t-0.0415719315814929\t-0.0356195506291120\t-0.0296671696767310\t-0.0237147887243500\t-0.0177624077719691\t-0.0118100268195881\t-0.00585764586720720\t0\t0.00585764586720720\t0.0118100268195881\t0.0177624077719691\t0.0237147887243500\t0.0296671696767310\t0.0356195506291120\t0.0415719315814929\t0.0475243125338739\t0.0534766934862548\t0.0594290744386358\t0.0653814553910168\t0.0713338363433977\t0.0772862172957787\t0.0832385982481596\t0.0891909792005406\t0.0951433601529216\t0.101095741105303\t0.107048122057683\t0.113000503010064\t0.118952883962445\t0.124905264914826\t0.130857645867207\t0.136810026819588\t0.142762407771969\t0.148714788724350\t0.154667169676731\t0.160619550629112\t0.166571931581493\t0.172524312533874\t0.178476693486255\t0.184429074438636\t0.190381455391017\t0.196333836343398\t0.202286217295779\t0.208238598248160\t0.214190979200541\t0.220143360152922\t0.226095741105303\t0.232048122057684\t0.238000503010065\t0.243952883962445\t0.249905264914826\t0.255857645867207\t0.261810026819588\t0.267762407771969\t0.273714788724350\t0.279667169676731\t0.285619550629112\t0.291571931581493\t0.297524312533874\t0.303476693486255\t0.309429074438636\t0.315381455391017\t0.321333836343398\t0.327286217295779\t0.333238598248160\t0.339190979200541\t0.345143360152921\t0.351095741105302\t0.357048122057683\t0.363000503010064\t0.368952883962445\t0.374905264914826\t0.380857645867207\t0.386810026819588\t0.392762407771969\t0.398714788724350\t0.404667169676731\t0.410619550629112\t0.416571931581493\t0.422524312533874\t0.428476693486255\t0.434429074438636\t0.440381455391017\t0.446333836343398\t0.452286217295779\t0.458238598248160\t0.464190979200541\t0.470143360152921\t0.476095741105302\t0.482048122057683\t0.488000503010064\t0.493952883962445\t0.499905264914826\t0.505857645867207\t0.511810026819588\t0.517762407771969\t0.523714788724350\t0.529667169676731\t0.535619550629112\t0.541571931581492]"  Table="[-9.10000000000000\t-9\t-8.90000000000000\t-8.80000000000000\t-8.70000000000000\t-8.60000000000000\t-8.50000000000000\t-8.40000000000000\t-8.30000000000000\t-8.20000000000000\t-8.10000000000000\t-8\t-7.90000000000000\t-7.80000000000000\t-7.70000000000000\t-7.60000000000000\t-7.50000000000000\t-7.40000000000000\t-7.30000000000000\t-7.20000000000000\t-7.10000000000000\t-7\t-6.90000000000000\t-6.80000000000000\t-6.70000000000000\t-6.60000000000000\t-6.50000000000000\t-6.40000000000000\t-6.30000000000000\t-6.20000000000000\t-6.10000000000000\t-6\t-5.90000000000000\t-5.80000000000000\t-5.70000000000000\t-5.60000000000000\t-5.50000000000000\t-5.40000000000000\t-5.30000000000000\t-5.20000000000000\t-5.10000000000000\t-5\t-4.90000000000000\t-4.80000000000000\t-4.70000000000000\t-4.60000000000000\t-4.50000000000000\t-4.40000000000000\t-4.30000000000000\t-4.20000000000000\t-4.10000000000000\t-4\t-3.90000000000000\t-3.80000000000000\t-3.70000000000000\t-3.60000000000000\t-3.50000000000000\t-3.40000000000000\t-3.30000000000000\t-3.20000000000000\t-3.10000000000000\t-3\t-2.90000000000000\t-2.80000000000000\t-2.70000000000000\t-2.60000000000000\t-2.50000000000000\t-2.40000000000000\t-2.30000000000000\t-2.20000000000000\t-2.10000000000000\t-2\t-1.90000000000000\t-1.80000000000000\t-1.70000000000000\t-1.60000000000000\t-1.50000000000000\t-1.40000000000000\t-1.30000000000000\t-1.20000000000000\t-1.10000000000000\t-1\t-0.900000000000000\t-0.800000000000000\t-0.700000000000000\t-0.600000000000000\t-0.500000000000000\t-0.400000000000000\t-0.300000000000000\t-0.200000000000000\t-0.100000000000000\t0\t0.100000000000000\t0.200000000000000\t0.300000000000000\t0.400000000000000\t0.500000000000000\t0.600000000000000\t0.700000000000000\t0.800000000000000\t0.900000000000000\t1\t1.10000000000000\t1.20000000000000\t1.30000000000000\t1.40000000000000\t1.50000000000000\t1.60000000000000\t1.70000000000000\t1.80000000000000\t1.90000000000000\t2\t2.10000000000000\t2.20000000000000\t2.30000000000000\t2.40000000000000\t2.50000000000000\t2.60000000000000\t2.70000000000000\t2.80000000000000\t2.90000000000000\t3\t3.10000000000000\t3.20000000000000\t3.30000000000000\t3.40000000000000\t3.50000000000000\t3.60000000000000\t3.70000000000000\t3.80000000000000\t3.90000000000000\t4\t4.10000000000000\t4.20000000000000\t4.30000000000000\t4.40000000000000\t4.50000000000000\t4.60000000000000\t4.70000000000000\t4.80000000000000\t4.90000000000000\t5\t5.10000000000000\t5.20000000000000\t5.30000000000000\t5.40000000000000\t5.50000000000000\t5.60000000000000\t5.70000000000000\t5.80000000000000\t5.90000000000000\t6\t6.10000000000000\t6.20000000000000\t6.30000000000000\t6.40000000000000\t6.50000000000000\t6.60000000000000\t6.70000000000000\t6.80000000000000\t6.90000000000000\t7\t7.10000000000000\t7.20000000000000\t7.30000000000000\t7.40000000000000\t7.50000000000000\t7.60000000000000\t7.70000000000000\t7.80000000000000\t7.90000000000000\t8\t8.10000000000000\t8.20000000000000\t8.30000000000000\t8.40000000000000\t8.50000000000000\t8.60000000000000\t8.70000000000000\t8.80000000000000\t8.90000000000000\t9\t9.10000000000000]"  InternalRulePriority=Speed  RndMeth=Simplest  InputSameDT=on
  Environment : Subsystem
  Monitor : Subsystem
  Steer : Constant  Value=0
  Step : Step  Time=5  After=0
  Switch : Switch  Criteria=u2 > Threshold
  Switch1 : Switch  Criteria=u2 > Threshold
  Switch2 : Switch  Criteria=u2 > Threshold
  To Workspace : ToWorkspace  VariableName=EvBoltCalib  SaveFormat=Structure With Time  SampleTime=-1
  Vector Concatenate : Concatenate  NumInputs=5
  Vehicle : Subsystem
  Out1 : Outport
  UseCarlaSpd : Outport  Port=2
  wires:
  Bus Creator2/1 -> Bus Selector/1, Monitor/1(Monitor)  "SimMonitor"
  [Driver] -> Bus Creator2/1  "Driver"
  Constant3/1 -> Bus Creator/4  "CltchCmd"
  Cmd/1 -> Demux/1
  Bus Creator/1 -> [Driver], Vehicle/2(Driver)
  Vehicle/1(Veh) -> Bus Creator2/2, [Veh]  "Veh"
  Environment/1(Env) -> Vehicle/1(Env)
  Constant/1 -> Environment/1(Grade)
  Constant4/1 -> Bus Creator/5  "lgSw"
  Bus Creator1/1 -> To Workspace/1
  Constant2/1 -> Bus Creator/3  "GearCmd"
  Vector Concatenate/1 -> Out1/1
  Clock/1 -> Vector Concatenate/4, Bus Creator1/8
  Bus Selector/1 -> Vector Concatenate/1, Bus Creator1/1  "<X>"
  Bus Selector/2 -> Vector Concatenate/2, Bus Creator1/2  "<Y>"
  Bus Selector/3 -> Vector Concatenate/3, Bus Creator1/3  "<psi>"
  Bus Selector/4 -> Bus Creator1/4  "<BattSoc>"
  Bus Selector/5 -> Bus Creator1/5  "<BattCurr>"
  Bus Selector/6 -> Bus Creator1/6  "<BattVolt>"
  Bus Selector/7 -> Bus Creator1/7  "<Axl1Trq>"
  Bus Selector/8 -> Vector Concatenate/5  "<VehSpd>"
  EV Bolt Steer/1 -> Bus Creator/6  "SteeringCmd"
  Switch2/1 -> EV Bolt Steer/1
  Switch/1 -> Bus Creator/1, AccelCmdOutput_Anye/1  "AccelCmd"
  Switch1/1 -> Bus Creator/2  "DecelCmd"
  Manual ot auto/1 -> [Autopilot]
  [Autopilot] -> Switch2/2, Switch1/2, Switch/2
  Step/1 -> Switch/3  "AccelCmd"
  Demux/1 -> Switch/1  "AccelCmd"
  Constant6/1 -> Switch1/3  "DecelCmd"
  Demux/2 -> Switch1/1  "DecelCmd"
  Steer/1 -> Switch2/3
  Demux/3 -> Switch2/1
  CarlaCmd/1 -> Vehicle/3(CarCmd)
  Vehicle/2(Output) -> UseCarlaSpd/1

== system CAVE_MachE_speedTrack0202/TCP SCALEXIO/ARE_First_Order_Derivative_[1,0,0]6 ==
  HDV_First_v : Inport
  Trigger : TriggerPort  TriggerType=either  VariantControl=Variant  ZeroCross=off  PortDimensions=1
  Constant : Constant  Value=0.01
  Constant1 : Constant  Value=13
  MATLAB Function : MATLAB Function  TreatAsAtomicUnit=on
  HDV_First_v_dot_hat : Outport  VectorParamsAs1DForOutWhenUnconnected=off
  wires:
  Constant1/1 -> MATLAB Function/3(u_init)
  HDV_First_v/1 -> MATLAB Function/1(U)
  MATLAB Function/1(Dot_U) -> HDV_First_v_dot_hat/1
  Constant/1 -> MATLAB Function/2(Ts)

== system CAVE_MachE_speedTrack0202/TCP SCALEXIO/Bytes2Double ==
  byte1 : Inport
  byte2 : Inport  Port=2
  byte3 : Inport  Port=3
  byte4 : Inport  Port=4
  Data Type Conversion2 : DataTypeConversion
  MATLAB Function2 : MATLAB Function  TreatAsAtomicUnit=on
  data : Outport
  wires:
  byte1/1 -> MATLAB Function2/1(byte1)
  byte3/1 -> MATLAB Function2/3(byte3)
  MATLAB Function2/1(float32) -> Data Type Conversion2/1
  byte4/1 -> MATLAB Function2/4(byte4)
  Data Type Conversion2/1 -> data/1
  byte2/1 -> MATLAB Function2/2(byte2)

== system CAVE_MachE_speedTrack0202/TCP SCALEXIO/Bytes2Double1 ==
  byte1 : Inport
  byte2 : Inport  Port=2
  byte3 : Inport  Port=3
  byte4 : Inport  Port=4
  Data Type Conversion2 : DataTypeConversion
  MATLAB Function2 : MATLAB Function  TreatAsAtomicUnit=on
  data : Outport
  wires:
  byte1/1 -> MATLAB Function2/1(byte1)
  byte3/1 -> MATLAB Function2/3(byte3)
  MATLAB Function2/1(float32) -> Data Type Conversion2/1
  byte4/1 -> MATLAB Function2/4(byte4)
  Data Type Conversion2/1 -> data/1
  byte2/1 -> MATLAB Function2/2(byte2)

== system CAVE_MachE_speedTrack0202/TCP SCALEXIO/Bytes2Double2 ==
  byte1 : Inport
  byte2 : Inport  Port=2
  byte3 : Inport  Port=3
  byte4 : Inport  Port=4
  Data Type Conversion2 : DataTypeConversion
  MATLAB Function2 : MATLAB Function  TreatAsAtomicUnit=on
  data : Outport
  wires:
  byte2/1 -> MATLAB Function2/2(byte2)
  Data Type Conversion2/1 -> data/1
  byte4/1 -> MATLAB Function2/4(byte4)
  MATLAB Function2/1(float32) -> Data Type Conversion2/1
  byte3/1 -> MATLAB Function2/3(byte3)
  byte1/1 -> MATLAB Function2/1(byte1)

== system CAVE_MachE_speedTrack0202/TCP SCALEXIO/Bytes2Double3 ==
  byte1 : Inport
  byte2 : Inport  Port=2
  byte3 : Inport  Port=3
  byte4 : Inport  Port=4
  Data Type Conversion2 : DataTypeConversion
  MATLAB Function2 : MATLAB Function  TreatAsAtomicUnit=on
  data : Outport
  wires:
  byte2/1 -> MATLAB Function2/2(byte2)
  Data Type Conversion2/1 -> data/1
  byte4/1 -> MATLAB Function2/4(byte4)
  MATLAB Function2/1(float32) -> Data Type Conversion2/1
  byte3/1 -> MATLAB Function2/3(byte3)
  byte1/1 -> MATLAB Function2/1(byte1)

== system CAVE_MachE_speedTrack0202/TCP SCALEXIO/Double2Bytes1 ==
  data : Inport
  MATLAB Function3 : MATLAB Function  TreatAsAtomicUnit=on
  Saturation : Saturate  UpperLimit=1e6  LowerLimit=-1e6
  byte1 : Outport
  byte2 : Outport  Port=2
  byte3 : Outport  Port=3
  byte4 : Outport  Port=4
  wires:
  Saturation/1 -> MATLAB Function3/1(defloatMe)
  MATLAB Function3/4(byte4) -> byte4/1
  MATLAB Function3/1(byte1) -> byte1/1
  MATLAB Function3/2(byte2) -> byte2/1
  data/1 -> Saturation/1
  MATLAB Function3/3(byte3) -> byte3/1

== system CAVE_MachE_speedTrack0202/TCP SCALEXIO/Subsystem9 ==
  dis_to_MP : Inport
  Add5 : Sum
  Compare To Constant1 : simulink/Logic and Bit Operations/Compare To Constant  relop=<=  const=150  OutDataTypeStr=boolean
  Compare To Constant2 : simulink/Logic and Bit Operations/Compare To Constant  relop=>  const=0  OutDataTypeStr=boolean
  Data Type Conversion : DataTypeConversion
  Delay : Delay  DelayLength=1
  Ctrl_enabled : Outport
  Ctrl_enable_Index : Outport  Port=2
  wires:
  Data Type Conversion/1 -> Add5/1
  Delay/1 -> Ctrl_enable_Index/1, Add5/2, Compare To Constant2/1
  Add5/1 -> Delay/1
  Compare To Constant2/1 -> Ctrl_enabled/1
  Compare To Constant1/1 -> Data Type Conversion/1
  dis_to_MP/1 -> Compare To Constant1/1

== system CAVE_MachE_speedTrack0202/TCP SCALEXIO/UlMPC ==
  note: Local (distributed) planning & control
      | based on the merging speed ref from RSU
  HDV_First_v_dot_hat : Inport
  v_ref : Inport  Port=2
  HDV_First_v : Inport  Port=3
  Enable : EnablePort
  BETA_HDV : Constant  Value=8
  CVXGEN_Leader_ULMPC_Spd_Ctrl_ : S-Function  Description=Simulink:masks:SFunctionBuilder_MD  InitFcn=try, set_param(gcb,'FunctionName','CVXGEN_Leader_Spd_ULMPC'), end  FunctionName=CVXGEN_Leader_Spd_ULMPC  SFunctionModules=CVXGEN_Leader_Spd_ULMPC_wrapper solver util matrix_support ldl  SFunctionDeploymentMode=off  EnableBusSupport=off
      mask init:
      | val = [[.9  0.75 0.75 1 1 .9 .9 1]',[1 1 0.75 0.75 .9 .9 1 .9]'];try , sys = get_param(gcb,'SfunBuilderFcnName');if isempty(sys), sys = get_param(gcb,'FunctionName'); end,catch, sys = get_param(gcb,'FunctionName'); end
      settings: CopyFcn=set_param(gcbh,'LinkStatus','none')  PreSaveFcn=try, set_param(gcb,'FunctionName','CVXGEN_Leader_Spd_ULMPC'), end  OpenFcn=sfunctionwizard(gcbh)
      mask Display: plot(val(:,1),val(:,2)),disp(sys), port_label('input',1,'vmax'), port_label('input',2,'vmin'), port_label('input',3,'deltav_max'), port_label('input',4,'deltav_min'), port_label('input',5,'vcmd_max'), port_label('input',6,'vcmd_min'), port_label('input',7,'delta_vcmd_max'), port_label('input',8,'delta_vcmd_min'), port_label('input',9,'A'), port_label('input',10,'B'), port_label('input',11,'d_k'), port_label('input',12,'Q'), port_label('input',13,'R'), port_label('input',14,'v_ref'), port_label('input',15,'v_cmd_last'), port_label('input',16,'x_0'), port_label('output',1,'delta_v_cmd_opt'), port_label('output',2,'v_cmd_opt')
  Constant54 : Constant  Value=0.05
  Constant55 : Constant  Value=-0.06
  Constant57 : Constant  Value=40
  Constant58 : Constant  Value=0
  Constant59 : Constant  Value=0.01
  Memory3 : Memory  InitialCondition=13  InheritSampleTime=on
  Q : Constant
  "R " : Constant  Value=20
  Rate Transition{6,48..50,68,70..80} (16 alike) : RateTransition
  Sys_Leader : MATLAB Function  TreatAsAtomicUnit=on
  Terminator : Terminator
  v_cmd_opt : Outport
  wires:
  Sys_Leader/1(A) -> Rate Transition71/1
  CVXGEN_Leader_ULMPC_Spd_Ctrl_/1 -> Terminator/1
  "R "/1 -> Rate Transition75/1
  Rate Transition68/1 -> CVXGEN_Leader_ULMPC_Spd_Ctrl_/3
  Constant57/1 -> Rate Transition49/1, Rate Transition73/1
  Rate Transition78/1 -> CVXGEN_Leader_ULMPC_Spd_Ctrl_/8
  Rate Transition72/1 -> CVXGEN_Leader_ULMPC_Spd_Ctrl_/10
  Constant54/1 -> Rate Transition68/1, Rate Transition77/1
  Rate Transition49/1 -> CVXGEN_Leader_ULMPC_Spd_Ctrl_/1
  Rate Transition77/1 -> CVXGEN_Leader_ULMPC_Spd_Ctrl_/7
  Rate Transition50/1 -> CVXGEN_Leader_ULMPC_Spd_Ctrl_/2
  BETA_HDV/1 -> Sys_Leader/2(beta)
  Rate Transition71/1 -> CVXGEN_Leader_ULMPC_Spd_Ctrl_/9
  Rate Transition75/1 -> CVXGEN_Leader_ULMPC_Spd_Ctrl_/13
  Rate Transition6/1 -> CVXGEN_Leader_ULMPC_Spd_Ctrl_/16
  Constant59/1 -> Sys_Leader/1(Ts)
  Rate Transition48/1 -> CVXGEN_Leader_ULMPC_Spd_Ctrl_/11
  HDV_First_v_dot_hat/1 -> Sys_Leader/3(v_dot_hat)
  Q/1 -> Rate Transition74/1
  CVXGEN_Leader_ULMPC_Spd_Ctrl_/2 -> v_cmd_opt/1, Memory3/1  "v_cmd_opt"
  HDV_First_v/1 -> Rate Transition6/1
  Rate Transition73/1 -> CVXGEN_Leader_ULMPC_Spd_Ctrl_/5
  Rate Transition79/1 -> CVXGEN_Leader_ULMPC_Spd_Ctrl_/14  "21"
  Sys_Leader/3(dk) -> Rate Transition48/1
  Rate Transition80/1 -> CVXGEN_Leader_ULMPC_Spd_Ctrl_/15
  Rate Transition70/1 -> CVXGEN_Leader_ULMPC_Spd_Ctrl_/4
  Rate Transition76/1 -> CVXGEN_Leader_ULMPC_Spd_Ctrl_/6
  Sys_Leader/2(B) -> Rate Transition72/1
  Constant55/1 -> Rate Transition70/1, Rate Transition78/1
  Memory3/1 -> Rate Transition80/1
  Constant58/1 -> Rate Transition50/1, Rate Transition76/1
  Rate Transition74/1 -> CVXGEN_Leader_ULMPC_Spd_Ctrl_/12
  v_ref/1 -> Rate Transition79/1

== system CAVE_MachE_speedTrack0202/Vehicle Under Test/Environment ==
  Grade : Inport
  Friction : Constant  Value=ones(4,1).*1
  Ground Feedback : Subsystem  VariantControlMode=Label  Variant=on  LabelModeActiveChoice=0
  Ground Z Level : Constant  Value=zeros(4,1)
  Subsystem : Subsystem
  Subsystem1 : Subsystem
      mask Display: disp('')
  Env : Outport
  wires:
  Subsystem/3(WindVel) -> Subsystem1/3(WindVel)
  Subsystem/2(EnvTemp) -> Subsystem1/2(EnvTemp)
  Subsystem/4(RoadGrade) -> Subsystem1/4(RoadGrade)
  Subsystem/1(EnvPrs) -> Subsystem1/1(EnvPrs)
  Subsystem1/1(Env) -> Env/1
  Friction/1 -> Ground Feedback/1(Friction)
  Ground Feedback/1(Ground) -> Subsystem1/5(GroundBus)  "Gnd"
  Ground Z Level/1 -> Ground Feedback/2(Ground Z Level)
  Grade/1 -> Subsystem/1(Grade)

== system CAVE_MachE_speedTrack0202/Vehicle Under Test/Monitor ==
  Monitor : Inport
  Calculate Fuel MPG : Subsystem  Commented=on
  Calculate Powertrain Energy : Subsystem
  Terminator : Terminator
  Terminator3 : Terminator
  wires:
  Calculate Fuel MPG/1(FuelEconMPG) -> Terminator/1  "FuelEconMpg"
  Monitor/1 -> Calculate Powertrain Energy/1(Monitor), Calculate Fuel MPG/1(Monitor)
  Calculate Powertrain Energy/1(TransEnrgyOutkWh) -> Terminator3/1  "DiffEnrgyInkWh"
